simulink library "MCA_lib"  (Simulink 7.5)
settings: Solver=ode45  StartTime=0.0  StopTime=10.0  RelTol=1e-3
undefined symbols (not defined in the file or in its folder): MotCtrlModTyp, p_bool_False_M, p_bool_True_M
libraries: BaseOperationLib_Browser x12, simulink x1
settings Model: Creator=wuaibin  LastModifiedBy=wuaibin

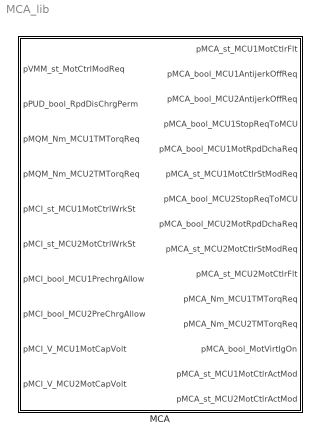
== system MCA_lib ==
  MCA : Subsystem  TreatAsAtomicUnit=on

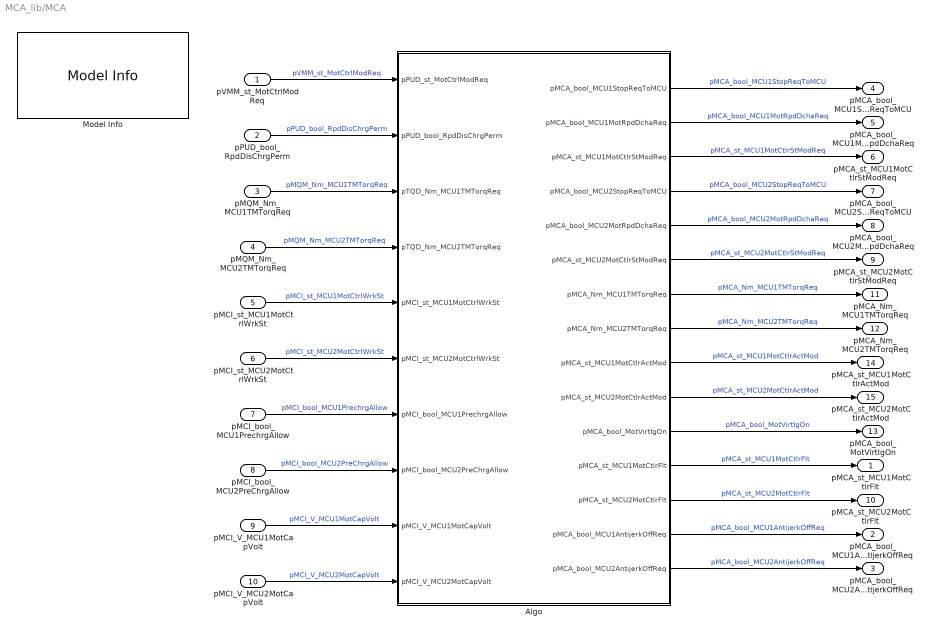
== system MCA_lib/MCA ==
  pVMM_st_MotCtrlModReq : Inport  OutDataType=fixdt(1, 16)  OutScaling=2^0
  pPUD_bool_RpdDisChrgPerm : Inport  Port=2  OutDataType=fixdt(1, 16)  OutScaling=2^0
  pMQM_Nm_MCU1TMTorqReq : Inport  Port=3  OutDataType=fixdt(1, 16)  OutScaling=2^0
  pMQM_Nm_MCU2TMTorqReq : Inport  Port=4  OutDataType=fixdt(1, 16)  OutScaling=2^0
  pMCI_st_MCU1MotCtrlWrkSt : Inport  Port=5  OutDataType=fixdt(1, 16)  OutScaling=2^0
  pMCI_st_MCU2MotCtrlWrkSt : Inport  Port=6  OutDataType=fixdt(1, 16)  OutScaling=2^0
  pMCI_bool_MCU1PrechrgAllow : Inport  Port=7  OutDataType=fixdt(1, 16)  OutScaling=2^0
  pMCI_bool_MCU2PreChrgAllow : Inport  Port=8
  pMCI_V_MCU1MotCapVolt : Inport  Port=9  OutDataType=fixdt(1, 16)  OutScaling=2^0
  pMCI_V_MCU2MotCapVolt : Inport  Port=10  OutDataType=fixdt(1, 16)  OutScaling=2^0
  Algo : Subsystem
  Model Info : simulink/Model-Wide Utilities/Model Info  SystemSampleTime=-1  InitialBlockCM=None  BlockCM=None  Frame=on  DisplayStringWithTags=Model Info\nCreated: %<Created>\nCreator: wuaibin  HorizontalTextAlignment=Center  LeftAlignmentValue=0.5  SourceBlockDiagram=HQEV_HCU  TagMaxNumber=20
  pMCA_st_MCU1MotCtlrFlt : Outport  OutDataType=fixdt(1, 16)  OutScaling=2^0
  pMCA_bool_MCU1AntijerkOffReq : Outport  Port=2
  pMCA_bool_MCU2AntijerkOffReq : Outport  Port=3
  pMCA_bool_MCU1StopReqToMCU : Outport  Port=4
  pMCA_bool_MCU1MotRpdDchaReq : Outport  Port=5
  pMCA_st_MCU1MotCtlrStModReq : Outport  Port=6
  pMCA_bool_MCU2StopReqToMCU : Outport  Port=7
  pMCA_bool_MCU2MotRpdDchaReq : Outport  Port=8
  pMCA_st_MCU2MotCtlrStModReq : Outport  Port=9
  pMCA_st_MCU2MotCtlrFlt : Outport  Port=10  OutDataType=fixdt(1, 16)  OutScaling=2^0
  pMCA_Nm_MCU1TMTorqReq : Outport  Port=11  OutDataType=fixdt(1, 16)  OutScaling=2^0
  pMCA_Nm_MCU2TMTorqReq : Outport  Port=12  OutDataType=fixdt(1, 16)  OutScaling=2^0
  pMCA_bool_MotVirtIgOn : Outport  Port=13
  pMCA_st_MCU1MotCtlrActMod : Outport  Port=14  OutDataType=fixdt(1, 16)  OutScaling=2^0
  pMCA_st_MCU2MotCtlrActMod : Outport  Port=15  OutDataType=fixdt(1, 16)  OutScaling=2^0
  wires:
  pPUD_bool_RpdDisChrgPerm/1 -> Algo/2(pPUD_bool_RpdDisChrgPerm)  "pPUD_bool_RpdDisChrgPerm"
  Algo/10(pMCA_st_MCU2MotCtlrActMod) -> pMCA_st_MCU2MotCtlrActMod/1  "pMCA_st_MCU2MotCtlrActMod"
  Algo/9(pMCA_st_MCU1MotCtlrActMod) -> pMCA_st_MCU1MotCtlrActMod/1  "pMCA_st_MCU1MotCtlrActMod"
  Algo/11(pMCA_bool_MotVirtIgOn) -> pMCA_bool_MotVirtIgOn/1  "pMCA_bool_MotVirtIgOn"
  pMQM_Nm_MCU2TMTorqReq/1 -> Algo/4(pTQD_Nm_MCU2TMTorqReq)  "pMQM_Nm_MCU2TMTorqReq"
  pMQM_Nm_MCU1TMTorqReq/1 -> Algo/3(pTQD_Nm_MCU1TMTorqReq)  "pMQM_Nm_MCU1TMTorqReq"
  Algo/8(pMCA_Nm_MCU2TMTorqReq) -> pMCA_Nm_MCU2TMTorqReq/1  "pMCA_Nm_MCU2TMTorqReq"
  Algo/7(pMCA_Nm_MCU1TMTorqReq) -> pMCA_Nm_MCU1TMTorqReq/1  "pMCA_Nm_MCU1TMTorqReq"
  pVMM_st_MotCtrlModReq/1 -> Algo/1(pPUD_st_MotCtrlModReq)  "pVMM_st_MotCtrlModReq"
  pMCI_st_MCU1MotCtrlWrkSt/1 -> Algo/5(pMCI_st_MCU1MotCtrlWrkSt)  "pMCI_st_MCU1MotCtrlWrkSt"
  pMCI_st_MCU2MotCtrlWrkSt/1 -> Algo/6(pMCI_st_MCU2MotCtrlWrkSt)  "pMCI_st_MCU2MotCtrlWrkSt"
  Algo/12(pMCA_st_MCU1MotCtlrFlt) -> pMCA_st_MCU1MotCtlrFlt/1  "pMCA_st_MCU1MotCtlrFlt"
  Algo/14(pMCA_bool_MCU1AntijerkOffReq) -> pMCA_bool_MCU1AntijerkOffReq/1  "pMCA_bool_MCU1AntijerkOffReq"
  Algo/15(pMCA_bool_MCU2AntijerkOffReq) -> pMCA_bool_MCU2AntijerkOffReq/1  "pMCA_bool_MCU2AntijerkOffReq"
  Algo/1(pMCA_bool_MCU1StopReqToMCU) -> pMCA_bool_MCU1StopReqToMCU/1  "pMCA_bool_MCU1StopReqToMCU"
  Algo/2(pMCA_bool_MCU1MotRpdDchaReq) -> pMCA_bool_MCU1MotRpdDchaReq/1  "pMCA_bool_MCU1MotRpdDchaReq"
  Algo/4(pMCA_bool_MCU2StopReqToMCU) -> pMCA_bool_MCU2StopReqToMCU/1  "pMCA_bool_MCU2StopReqToMCU"
  Algo/5(pMCA_bool_MCU2MotRpdDchaReq) -> pMCA_bool_MCU2MotRpdDchaReq/1  "pMCA_bool_MCU2MotRpdDchaReq"
  Algo/3(pMCA_st_MCU1MotCtlrStModReq) -> pMCA_st_MCU1MotCtlrStModReq/1  "pMCA_st_MCU1MotCtlrStModReq"
  Algo/6(pMCA_st_MCU2MotCtlrStModReq) -> pMCA_st_MCU2MotCtlrStModReq/1  "pMCA_st_MCU2MotCtlrStModReq"
  Algo/13(pMCA_st_MCU2MotCtlrFlt) -> pMCA_st_MCU2MotCtlrFlt/1  "pMCA_st_MCU2MotCtlrFlt"
  pMCI_bool_MCU1PrechrgAllow/1 -> Algo/7(pMCI_bool_MCU1PrechrgAllow)  "pMCI_bool_MCU1PrechrgAllow"
  pMCI_bool_MCU2PreChrgAllow/1 -> Algo/8(pMCI_bool_MCU2PreChrgAllow)  "pMCI_bool_MCU2PreChrgAllow"
  pMCI_V_MCU1MotCapVolt/1 -> Algo/9(pMCI_V_MCU1MotCapVolt)  "pMCI_V_MCU1MotCapVolt"
  pMCI_V_MCU2MotCapVolt/1 -> Algo/10(pMCI_V_MCU2MotCapVolt)  "pMCI_V_MCU2MotCapVolt"

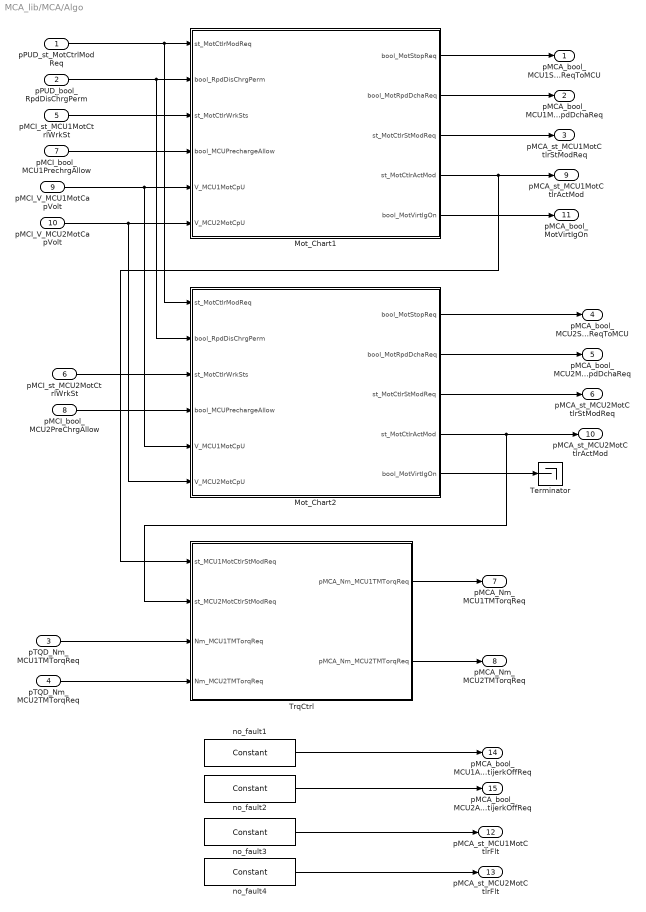
== system MCA_lib/MCA/Algo ==
  pPUD_st_MotCtrlModReq : Inport  OutDataType=fixdt(1, 16)  OutScaling=2^0
  pPUD_bool_RpdDisChrgPerm : Inport  Port=2  OutDataType=fixdt(1, 16)  OutScaling=2^0
  pTQD_Nm_MCU1TMTorqReq : Inport  Port=3  OutDataType=fixdt(1, 16)  OutScaling=2^0
  pTQD_Nm_MCU2TMTorqReq : Inport  Port=4  OutDataType=fixdt(1, 16)  OutScaling=2^0
  pMCI_st_MCU1MotCtrlWrkSt : Inport  Port=5  OutDataType=fixdt(1, 16)  OutScaling=2^0
  pMCI_st_MCU2MotCtrlWrkSt : Inport  Port=6  OutDataType=fixdt(1, 16)  OutScaling=2^0
  pMCI_bool_MCU1PrechrgAllow : Inport  Port=7  OutDataType=fixdt(1, 16)  OutScaling=2^0
  pMCI_bool_MCU2PreChrgAllow : Inport  Port=8
  pMCI_V_MCU1MotCapVolt : Inport  Port=9  OutDataType=fixdt(1, 16)  OutScaling=2^0
  pMCI_V_MCU2MotCapVolt : Inport  Port=10  OutDataType=fixdt(1, 16)  OutScaling=2^0
  Mot_Chart1 : Stateflow chart  TreatAsAtomicUnit=on
  Mot_Chart2 : Stateflow chart  TreatAsAtomicUnit=on
  Terminator : Terminator
  TrqCtrl : Subsystem
  no_fault1 : BaseOperationLib_Browser/Sources&Sinks/Constant  Value=p_bool_True_M  OutMin=[]  OutMax=[]  OutDataType=fixdt(1, 16)  ConRadixGroup=Use specified scaling  OutScaling=2^0  OutDataTypeStr=Inherit: Inherit via back propagation
  no_fault2 : BaseOperationLib_Browser/Sources&Sinks/Constant  Value=p_bool_True_M  OutMin=[]  OutMax=[]  OutDataType=fixdt(1, 16)  ConRadixGroup=Use specified scaling  OutScaling=2^0  OutDataTypeStr=Inherit: Inherit via back propagation
  no_fault3 : BaseOperationLib_Browser/Sources&Sinks/Constant  Value=p_bool_False_M  OutMin=[]  OutMax=[]  OutDataType=fixdt(1, 16)  ConRadixGroup=Use specified scaling  OutScaling=2^0  OutDataTypeStr=Inherit: Inherit via back propagation
  no_fault4 : BaseOperationLib_Browser/Sources&Sinks/Constant  Value=p_bool_False_M  OutMin=[]  OutMax=[]  OutDataType=fixdt(1, 16)  ConRadixGroup=Use specified scaling  OutScaling=2^0  OutDataTypeStr=Inherit: Inherit via back propagation
  pMCA_bool_MCU1StopReqToMCU : Outport
  pMCA_bool_MCU1MotRpdDchaReq : Outport  Port=2
  pMCA_st_MCU1MotCtlrStModReq : Outport  Port=3
  pMCA_bool_MCU2StopReqToMCU : Outport  Port=4
  pMCA_bool_MCU2MotRpdDchaReq : Outport  Port=5
  pMCA_st_MCU2MotCtlrStModReq : Outport  Port=6
  pMCA_Nm_MCU1TMTorqReq : Outport  Port=7  OutDataType=fixdt(1, 16)  OutScaling=2^0
  pMCA_Nm_MCU2TMTorqReq : Outport  Port=8  OutDataType=fixdt(1, 16)  OutScaling=2^0
  pMCA_st_MCU1MotCtlrActMod : Outport  Port=9  OutDataType=fixdt(1, 16)  OutScaling=2^0
  pMCA_st_MCU2MotCtlrActMod : Outport  Port=10  OutDataType=fixdt(1, 16)  OutScaling=2^0
  pMCA_bool_MotVirtIgOn : Outport  Port=11  OutDataType=fixdt(1, 16)  OutScaling=2^0
  pMCA_st_MCU1MotCtlrFlt : Outport  Port=12  OutDataType=fixdt(1, 16)  OutScaling=2^0
  pMCA_st_MCU2MotCtlrFlt : Outport  Port=13  OutDataType=fixdt(1, 16)  OutScaling=2^0
  pMCA_bool_MCU1AntijerkOffReq : Outport  Port=14
  pMCA_bool_MCU2AntijerkOffReq : Outport  Port=15
  wires:
  Mot_Chart2/3(st_MotCtlrStModReq) -> pMCA_st_MCU2MotCtlrStModReq/1
  Mot_Chart2/5(bool_MotVirtIgOn) -> Terminator/1
  Mot_Chart2/4(st_MotCtlrActMod) -> pMCA_st_MCU2MotCtlrActMod/1, TrqCtrl/2(st_MCU2MotCtlrStModReq)
  Mot_Chart1/5(bool_MotVirtIgOn) -> pMCA_bool_MotVirtIgOn/1
  no_fault2/1 -> pMCA_bool_MCU2AntijerkOffReq/1
  no_fault1/1 -> pMCA_bool_MCU1AntijerkOffReq/1
  pPUD_bool_RpdDisChrgPerm/1 -> Mot_Chart1/2(bool_RpdDisChrgPerm), Mot_Chart2/2(bool_RpdDisChrgPerm)
  TrqCtrl/2(pMCA_Nm_MCU2TMTorqReq) -> pMCA_Nm_MCU2TMTorqReq/1
  pTQD_Nm_MCU2TMTorqReq/1 -> TrqCtrl/4(Nm_MCU2TMTorqReq)
  TrqCtrl/1(pMCA_Nm_MCU1TMTorqReq) -> pMCA_Nm_MCU1TMTorqReq/1
  pTQD_Nm_MCU1TMTorqReq/1 -> TrqCtrl/3(Nm_MCU1TMTorqReq)
  pPUD_st_MotCtrlModReq/1 -> Mot_Chart1/1(st_MotCtlrModReq), Mot_Chart2/1(st_MotCtlrModReq)
  pMCI_st_MCU1MotCtrlWrkSt/1 -> Mot_Chart1/3(st_MotCtlrWrkSts)
  pMCI_st_MCU2MotCtrlWrkSt/1 -> Mot_Chart2/3(st_MotCtlrWrkSts)
  Mot_Chart2/1(bool_MotStopReq) -> pMCA_bool_MCU2StopReqToMCU/1
  Mot_Chart2/2(bool_MotRpdDchaReq) -> pMCA_bool_MCU2MotRpdDchaReq/1
  Mot_Chart1/1(bool_MotStopReq) -> pMCA_bool_MCU1StopReqToMCU/1
  Mot_Chart1/2(bool_MotRpdDchaReq) -> pMCA_bool_MCU1MotRpdDchaReq/1
  Mot_Chart1/3(st_MotCtlrStModReq) -> pMCA_st_MCU1MotCtlrStModReq/1
  Mot_Chart1/4(st_MotCtlrActMod) -> TrqCtrl/1(st_MCU1MotCtlrStModReq), pMCA_st_MCU1MotCtlrActMod/1
  pMCI_bool_MCU1PrechrgAllow/1 -> Mot_Chart1/4(bool_MCUPrechargeAllow)
  pMCI_bool_MCU2PreChrgAllow/1 -> Mot_Chart2/4(bool_MCUPrechargeAllow)
  pMCI_V_MCU1MotCapVolt/1 -> Mot_Chart1/5(V_MCU1MotCpU), Mot_Chart2/5(V_MCU1MotCpU)
  pMCI_V_MCU2MotCapVolt/1 -> Mot_Chart1/6(V_MCU2MotCpU), Mot_Chart2/6(V_MCU2MotCpU)
  no_fault3/1 -> pMCA_st_MCU1MotCtlrFlt/1
  no_fault4/1 -> pMCA_st_MCU2MotCtlrFlt/1

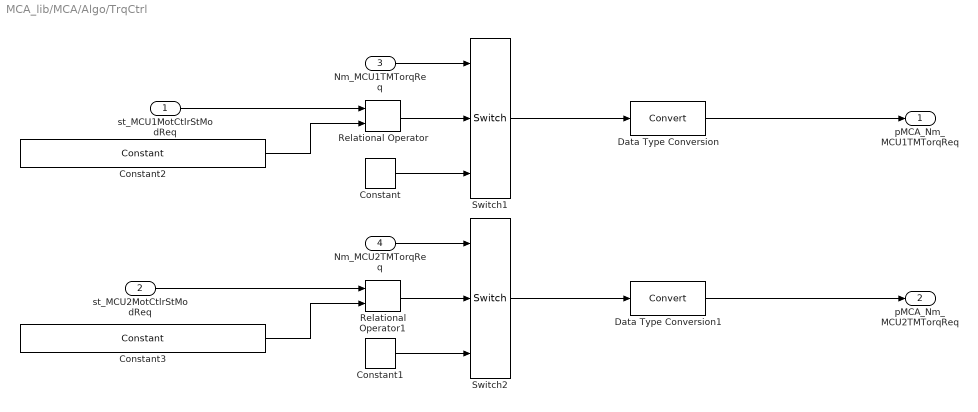
== system MCA_lib/MCA/Algo/TrqCtrl ==
  st_MCU1MotCtlrStModReq : Inport  OutDataType=fixdt(1, 16)  OutScaling=2^0
  st_MCU2MotCtlrStModReq : Inport  Port=2  OutDataType=fixdt(1, 16)  OutScaling=2^0
  Nm_MCU1TMTorqReq : Inport  Port=3  OutDataType=fixdt(1, 16)  OutScaling=2^0
  Nm_MCU2TMTorqReq : Inport  Port=4  OutDataType=fixdt(1, 16)  OutScaling=2^0
  Constant : BaseOperationLib_Browser/Sources&Sinks/Constant  Value=0  OutMin=[]  OutMax=[]  OutDataTypeMode=single  OutDataType=fixdt(1, 16)  ConRadixGroup=Use specified scaling  OutScaling=2^0  OutDataTypeStr=single
  Constant1 : BaseOperationLib_Browser/Sources&Sinks/Constant  Value=0  OutMin=[]  OutMax=[]  OutDataTypeMode=single  OutDataType=fixdt(1, 16)  ConRadixGroup=Use specified scaling  OutScaling=2^0  OutDataTypeStr=single
  Constant2 : BaseOperationLib_Browser/Sources&Sinks/Constant  Value=uint8(MotCtrlModTyp.MTC_TQ_IDLE)  OutMin=[]  OutMax=[]  OutDataType=fixdt(1, 16)  ConRadixGroup=Use specified scaling  OutScaling=2^0  OutDataTypeStr=Inherit: Inherit from 'Constant value'
  Constant3 : BaseOperationLib_Browser/Sources&Sinks/Constant  Value=uint8(MotCtrlModTyp.MTC_TQ_IDLE)  OutMin=[]  OutMax=[]  OutDataType=fixdt(1, 16)  ConRadixGroup=Use specified scaling  OutScaling=2^0  OutDataTypeStr=Inherit: Inherit from 'Constant value'
  Data Type Conversion : DataTypeConversion  OutDataType=fixdt(1, 16)  OutScaling=2^0
  Data Type Conversion1 : DataTypeConversion  OutDataType=fixdt(1, 16)  OutScaling=2^0
  Relational Operator : BaseOperationLib_Browser/Logic Operations Changed/Relational Operator  Operator===  InputSameDT=on  LogicOutDataTypeMode=Specify via dialog  LogicDataType=PDT_Bool  OutDataTypeStr=PDT_Bool
  Relational Operator1 : BaseOperationLib_Browser/Logic Operations Changed/Relational Operator  Operator===  InputSameDT=on  LogicOutDataTypeMode=Specify via dialog  LogicDataType=PDT_Bool  OutDataTypeStr=PDT_Bool
  Switch1 : BaseOperationLib_Browser/Signal Routing Changed/Switch  Criteria=u2 ~= 0  Threshold=1  InputSameDT=on  OutMin=[]  OutMax=[]  OutDataType=fixdt(1,16,0)  OutScaling=[]  SaturateOnIntegerOverflow=on
  Switch2 : BaseOperationLib_Browser/Signal Routing Changed/Switch  Criteria=u2 ~= 0  Threshold=1  InputSameDT=on  OutMin=[]  OutMax=[]  OutDataType=fixdt(1,16,0)  OutScaling=[]  SaturateOnIntegerOverflow=on
  pMCA_Nm_MCU1TMTorqReq : Outport  OutDataType=fixdt(1, 16)  OutScaling=2^0
  pMCA_Nm_MCU2TMTorqReq : Outport  Port=2  OutDataType=fixdt(1, 16)  OutScaling=2^0
  wires:
  Constant3/1 -> Relational Operator1/2
  st_MCU2MotCtlrStModReq/1 -> Relational Operator1/1
  Relational Operator1/1 -> Switch2/2
  Constant2/1 -> Relational Operator/2
  Relational Operator/1 -> Switch1/2
  st_MCU1MotCtlrStModReq/1 -> Relational Operator/1
  Constant1/1 -> Switch2/3
  Constant/1 -> Switch1/3
  Switch2/1 -> Data Type Conversion1/1
  Nm_MCU2TMTorqReq/1 -> Switch2/1
  Nm_MCU1TMTorqReq/1 -> Switch1/1
  Switch1/1 -> Data Type Conversion/1
  Data Type Conversion1/1 -> pMCA_Nm_MCU2TMTorqReq/1
  Data Type Conversion/1 -> pMCA_Nm_MCU1TMTorqReq/1

== stateflow chart MCA/Algo/Mot_Chart2 ==
  state Normal
    en:
    bool_MotVirtIgOn = true;
    bool_MotStopReq = false;
    bool_MotRpdDchaReq = false;
    state Initial
      en:
      st_MotCtlrStModReq = MotCtlrStsModTyp.NO_REQUEST;
      state Init
        en:
        st_MotCtlrActMod = MotCtrlModTyp.MTC_INIT;
      (default) -> Normal.Initial.Init
    state Standby_state
      en:
      st_MotCtlrStModReq = MotCtlrStsModTyp.NO_REQUEST;
      state Init
      state Standby
        en:
        st_MotCtlrActMod = MotCtrlModTyp.MTC_STANDBY;
      (default) -> Normal.Standby_state.Init
      Normal.Standby_state.Init -> Standby : [bool_MCUPrechargeAllow == true]
    state Torque_state
      en:
      st_MotCtlrStModReq = MotCtlrStsModTyp.TORQUE_MODE_REQUEST;
      state Init
      state TorqCtrl
        en:
        st_MotCtlrActMod = MotCtrlModTyp.MTC_TQ_IDLE;
      (default) -> Normal.Torque_state.Init
      Normal.Torque_state.Init -> TorqCtrl : [st_MotCtlrWrkSts == MotCtrlWrkStsTyp.MCWS_TORQUE_CONTROL]
    Initial -> Standby_state [order 1] : [st_MotCtlrModReq == MotCtrlModTyp.MTC_STANDBY]
    (default) -> Initial
    Standby_state -> Torque_state : [st_MotCtlrModReq == MotCtrlModTyp.MTC_TQ_IDLE]
    Initial -> Torque_state [order 2] : [st_MotCtlrModReq == MotCtrlModTyp.MTC_TQ_IDLE]
    Torque_state -> Standby_state : [st_MotCtlrModReq == MotCtrlModTyp.MTC_STANDBY]
  state stop_state
    en:
    bool_MotVirtIgOn = true;
    bool_MotStopReq = true;
    st_MotCtlrStModReq = MotCtlrStsModTyp.NO_REQUEST;
    state Init
      en:
      st_MotCtlrActMod = MotCtrlModTyp.MTC_STOP
    state Rapid_discharge
      en:
      bool_MotRpdDchaReq = true;
    (default) -> stop_state.Init
    stop_state.Init -> stop_state.Rapid_discharge : [bool_RpdDisChrgPerm == true]
  state shutdown_state
    en:
    bool_MotStopReq = true;
    bool_MotVirtIgOn = false;
    st_MotCtlrStModReq = MotCtlrStsModTyp.NO_REQUEST;
    state Init
      en:
      st_MotCtlrActMod = MotCtrlModTyp.MTC_SHUTDOWN;
    state Rapid_discharge
      en:
      bool_MotRpdDchaReq = true;
    (default) -> shutdown_state.Init
    shutdown_state.Init -> shutdown_state.Rapid_discharge : [bool_RpdDisChrgPerm == true]
  (default) -> Normal
  Normal -> stop_state [order 1] : [st_MotCtlrModReq == MotCtrlModTyp.MTC_STOP]
  stop_state -> Normal [order 2] : [st_MotCtlrModReq != MotCtrlModTyp.MTC_STOP]
  stop_state -> shutdown_state [order 1] : [st_MotCtlrModReq == MotCtrlModTyp.MTC_SHUTDOWN]
  Normal -> shutdown_state [order 2] : [st_MotCtlrModReq == MotCtrlModTyp.MTC_SHUTDOWN]
  shutdown_state -> Normal : [st_MotCtlrModReq != MotCtrlModTyp.MTC_SHUTDOWN]
  data: st_MotCtlrModReq input double; bool_RpdDisChrgPerm input double; bool_MotStopReq output boolean; bool_MotRpdDchaReq output boolean; st_MotCtlrStModReq output uint8; st_MotCtlrActMod output uint8; st_MotCtlrWrkSts input double; bool_MCUPrechargeAllow input double; V_MCU1MotCpU input double; V_MCU2MotCpU input double; bool_MotVirtIgOn output boolean

== stateflow chart MCA/Algo/Mot_Chart1 ==
  state Normal
    en:
    bool_MotVirtIgOn = true;
    bool_MotStopReq = false;
    bool_MotRpdDchaReq = false;
    state Initial
      en:
      st_MotCtlrStModReq = MotCtlrStsModTyp.NO_REQUEST;
      state Init
        en:
        st_MotCtlrActMod = MotCtrlModTyp.MTC_INIT;
      (default) -> Normal.Initial.Init
    state Standby_state
      en:
      st_MotCtlrStModReq = MotCtlrStsModTyp.NO_REQUEST;
      state Init
      state Standby
        en:
        st_MotCtlrActMod = MotCtrlModTyp.MTC_STANDBY;
      (default) -> Normal.Standby_state.Init
      Normal.Standby_state.Init -> Standby : [bool_MCUPrechargeAllow == true]
    state Torque_state
      en:
      st_MotCtlrStModReq = MotCtlrStsModTyp.TORQUE_MODE_REQUEST;
      state Init
      state TorqCtrl
        en:
        st_MotCtlrActMod = MotCtrlModTyp.MTC_TQ_IDLE;
      (default) -> Normal.Torque_state.Init
      Normal.Torque_state.Init -> TorqCtrl : [st_MotCtlrWrkSts == MotCtrlWrkStsTyp.MCWS_TORQUE_CONTROL]
    Initial -> Standby_state [order 1] : [st_MotCtlrModReq == MotCtrlModTyp.MTC_STANDBY]
    (default) -> Initial
    Standby_state -> Torque_state : [st_MotCtlrModReq == MotCtrlModTyp.MTC_TQ_IDLE]
    Initial -> Torque_state [order 2] : [st_MotCtlrModReq == MotCtrlModTyp.MTC_TQ_IDLE]
    Torque_state -> Standby_state : [st_MotCtlrModReq == MotCtrlModTyp.MTC_STANDBY]
  state stop_state
    en:
    bool_MotVirtIgOn = true;
    bool_MotStopReq = true;
    st_MotCtlrStModReq = MotCtlrStsModTyp.NO_REQUEST;
    state Init
      en:
      st_MotCtlrActMod = MotCtrlModTyp.MTC_STOP;
    state Rapid_dischargeEn
      en:
      bool_MotRpdDchaReq = true;
    (default) -> stop_state.Init
    stop_state.Init -> Rapid_dischargeEn : [bool_RpdDisChrgPerm == true]
  state shutdown_state
    en:
    bool_MotStopReq = true;
    bool_MotVirtIgOn = false;
    st_MotCtlrStModReq = MotCtlrStsModTyp.NO_REQUEST;
    state Init
      en:
      st_MotCtlrActMod = MotCtrlModTyp.MTC_SHUTDOWN;
    state Rapid_discharge
      en:
      bool_MotRpdDchaReq = true;
    (default) -> shutdown_state.Init
    shutdown_state.Init -> Rapid_discharge : [bool_RpdDisChrgPerm == true]
  (default) -> Normal
  Normal -> stop_state [order 1] : [st_MotCtlrModReq == MotCtrlModTyp.MTC_STOP]
  stop_state -> Normal [order 2] : [st_MotCtlrModReq != MotCtrlModTyp.MTC_STOP]
  stop_state -> shutdown_state [order 1] : [st_MotCtlrModReq == MotCtrlModTyp.MTC_SHUTDOWN]
  Normal -> shutdown_state [order 2] : [st_MotCtlrModReq == MotCtrlModTyp.MTC_SHUTDOWN]
  shutdown_state -> Normal : [st_MotCtlrModReq != MotCtrlModTyp.MTC_SHUTDOWN]
  data: st_MotCtlrModReq input double; bool_RpdDisChrgPerm input double; bool_MotStopReq output boolean; bool_MotRpdDchaReq output boolean; st_MotCtlrStModReq output uint8; st_MotCtlrActMod output uint8; st_MotCtlrWrkSts input double; bool_MCUPrechargeAllow input double; V_MCU1MotCpU input double; V_MCU2MotCpU input double; bool_MotVirtIgOn output boolean
